simulink model "cruise_control_identificacao"  (R2019b)
settings: Solver=VariableStepAuto  StartTime=0.0  StopTime=100.0  RelTol=1e-3
values from neighbouring files (symbols this model uses):
  a = load('data.mat')    [simulacoes.m]
  b = b + 10    [simulacoes.m]
undefined symbols (not defined in the file or in its folder): m
settings Model: Creator=rodri  LastModifiedBy=rodri

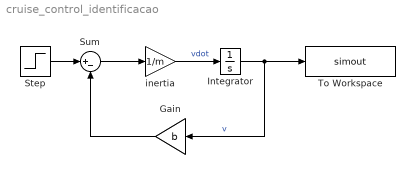
== system cruise_control_identificacao ==
  Gain : Gain  Gain=b
  Integrator : Integrator
  Step : Step  Time=0  After=a.data.f  SampleTime=0
  Sum : Sum  Inputs=|+-
  To Workspace : ToWorkspace  VariableName=simout  SaveFormat=Structure With Time  SampleTime=-1
  inertia : Gain  Gain=1/m
  wires:
  Integrator/1 -> To Workspace/1, Gain/1  "v"
  inertia/1 -> Integrator/1  "vdot"
  Sum/1 -> inertia/1
  Gain/1 -> Sum/2
  Step/1 -> Sum/1
